simulink model "DC_Motor"  (R2013a)
settings: Solver=ode45  StartTime=0.0  StopTime=30  RelTol=1e-3
settings Model: Creator=Admin  LastModifiedBy=Admin

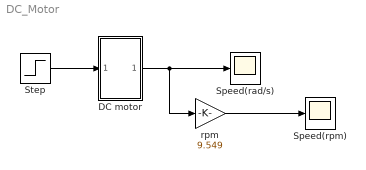
== system DC_Motor ==
  DC motor : Subsystem
  Speed(rad/s) : Scope
  Speed(rpm) : Scope
      settings: YMin=2256.6  YMax=2494.14
  Step : Step  Time=0  After=500  SampleTime=0
  rpm : Gain  Gain=9.549
  wires:
  rpm/1 -> Speed(rpm)/1
  DC motor/1(Out1) -> rpm/1, Speed(rad/s)/1
  Step/1 -> DC motor/1(In1)

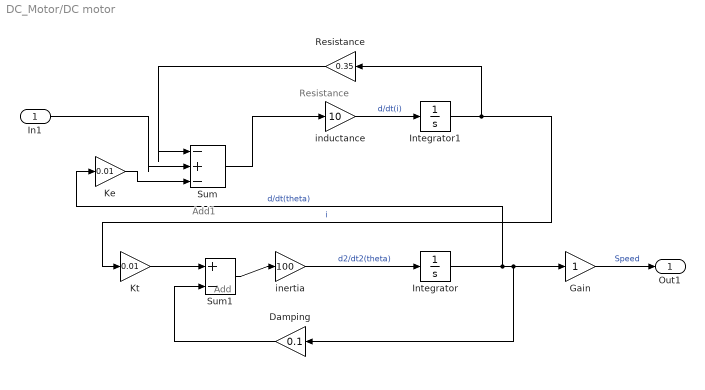
== system DC_Motor/DC motor ==
  note: Resistance
  note: Add
  note: Add1
  In1 : Inport
  Damping : Gain  Gain=0.1
  Gain : Gain
  Integrator : Integrator
  Integrator1 : Integrator
  Ke : Gain  Gain=0.01
  Kt : Gain  Gain=0.01
  Resistance : Gain  Gain=0.35
      settings: AttributesFormatString=Resistance
  Sum : Sum  Inputs=|-+-
  Sum1 : Sum  Inputs=|+-
  inductance : Gain  Gain=10
      settings: AttributesFormatString=1/L
  inertia : Gain  Gain=100
      settings: AttributesFormatString=1/J
  Out1 : Outport
  wires:
  Kt/1 -> Sum1/1
  Damping/1 -> Sum1/2
  Sum1/1 -> inertia/1
  inertia/1 -> Integrator/1  "d2/dt2(theta)"
  Integrator1/1 -> Resistance/1, Kt/1  "i"
  Ke/1 -> Sum/3
  Resistance/1 -> Sum/1
  Sum/1 -> inductance/1
  inductance/1 -> Integrator1/1  "d/dt(i)"
  Gain/1 -> Out1/1  "Speed"
  Integrator/1 -> Gain/1, Damping/1, Ke/1  "d/dt(theta)"
  In1/1 -> Sum/2
